simulink model "ESC251_MATLABTakeHome_Q1BD"  (R2025b)
settings: Solver=VariableStepAuto  StartTime=0.0  StopTime=0.5  RelTol=1e-3
values from neighbouring files (symbols this model uses):
  B = [0 ... (first row only)    [ESC251_HW4.m]    (also in ESC251_LabAssign.m = 0.01; ESC251_TakeHomeQ1.m = 0.01)
  Jeqb = (N^2)*J1b + J2b    (= 3.489856e-05)    [ESC251_LabAssign.m]    (also in ESC251_TakeHomeQ1.m)
  Kgb = Kmb    (= 0.042)    [ESC251_LabAssign.m]    (also in ESC251_TakeHomeQ1.m)
  Kmb = 0.042    [ESC251_LabAssign.m]    (also in ESC251_TakeHomeQ1.m)
  L = 0.1    [ESC251_LabAssign.m]    (also in ESC251_TakeHomeQ1.m; SystemsFinalProject_linearized_ramp.m = 1.1)
  N = 2    [ESC251_LabAssign.m]    (also in ESC251_TakeHomeQ1.m)
  Rb = 8.4    [ESC251_LabAssign.m]    (also in ESC251_TakeHomeQ1.m)
  s = tf('s')    [ESC251_HW8b.m]
undefined symbols (not defined in the file or in its folder): G
settings Model: Creator=mydkm  LastModifiedBy=mydkm

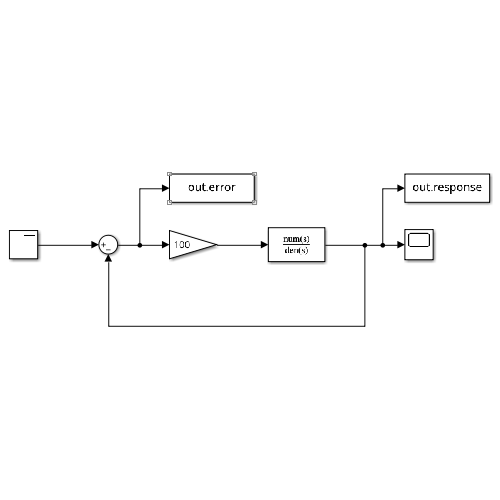
[thumbnail: Simulink's stored preview of the top-level diagram]
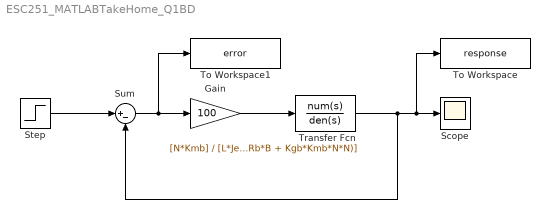
== system ESC251_MATLABTakeHome_Q1BD ==
  Gain : Gain  Gain=100
  Scope : Scope
  Step : Step  Time=0  SampleTime=0
  Sum : Sum  Inputs=|+-
  To Workspace : ToWorkspace  VariableName=response  SaveFormat=Timeseries  SampleTime=-1
  To Workspace1 : ToWorkspace  VariableName=error  SaveFormat=Timeseries  SampleTime=-1
  Transfer Fcn : TransferFcn  Numerator=[N*Kmb]  Denominator=[L*Jeqb, (B*L + Rb*Jeqb), (Rb*B + Kgb*Kmb*N*N)]  ContinuousStateAttributes=G(s)
  wires:
  Step/1 -> Sum/1
  Sum/1 -> To Workspace1/1, Gain/1
  Gain/1 -> Transfer Fcn/1
  Transfer Fcn/1 -> Sum/2, To Workspace/1, Scope/1
